simulink library "microCHP_modulating"  (R2018b)
settings: Solver=ode45  StartTime=0.0  StopTime=10.0  RelTol=1e-3  EnableMultiTasking=on
undefined symbols (not defined in the file): path_carnot
libraries: carnot x10
settings Model: Creator=lena.frank  LastModifiedBy=P41573
settings DataIOCC: LimitDataPoints=on  SaveFormat=Array  SignalLoggingSaveFormat=ModelDataLogs
settings OptimizationCC: ExpressionDepthLimit=2147483647  LifeSpan=inf
settings DebuggingCC: UnderspecifiedInitializationDetection=Classic  MergeDetectMultiDrivingBlocksExec=none  SolverPrmCheckMsg=warning  FcnCallInpInsideContextMsg=warning  StateNameClashWarn=warning  SFUnexpectedBacktrackingDiag=warning  SFNoUnconditionalDefaultTransitionDiag=warning  SFExecutionAtInitializationDiag=none
settings HardwareCC: ProdBitPerPointer=32  ProdBitPerSizeT=32  ProdBitPerPtrDiffT=32  ProdLargestAtomicFloat=None  ProdIntDivRoundTo=Undefined  ProdEndianess=Unspecified  ProdWordSize=32  ProdHWDeviceType=32-bit Generic
settings ModelReferenceCC: PropagateSignalLabelsOutOfModel=off
settings SFSimCC: SimUseLocalCustomCode=off
settings RTWCC: RTWUseLocalCustomCode=off
settings CodeAppCC: StateflowObjectComments=on
settings GRTTargetCC: TargetLangStandard=C89/C90 (ANSI)  GeneratePreprocessorConditionals=Disable all  CombineOutputUpdateFcns=off  GRTInterface=on
settings ConfigComp: CovMetricSettings=dw  CovHtmlReporting=on  CovSaveCumulativeToWorkspaceVar=on  CovSaveSingleToWorkspaceVar=on  CovExternalEMLEnable=off

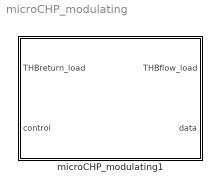
== system microCHP_modulating ==
  microCHP_modulating1 : Subsystem  mask(CHP){P_th_max=12500, P_th_min=3500, P_th_start=8000, f_P_el=0.37, T_flow_setpoint=80, T_flow_max=88, t_start=180, t_readjustment=450}
      mask prompts: P_th_max "maximum heating power [W]"; P_th_min "minimum heating power [W]"; P_th_start "initial heating power at start-up phase [W]"; f_P_el "electrical power fraction (referring to heating power) [0..1]"; T_flow_setpoint "flow setpoint temperature [°C]"; T_flow_max "maximum flow temperature [°C]"; t_start "duration of start-up phase [s]"; t_readjustment "duration of readjustment intervall [s]"
      mask help:
      | engine speed = f(T_return_load, T_flow_setpoint, T_flow, T_return)
      | T_return_load: a storage temperature or the return flow temperature.
      | Adjustable start-up phase: initial heating power
      | Ramp-up phase: maximum heating power up to 60°C
      | Control phase: heating power is readjusted after an inputed readjustment intervall.
      |
      | Return temperature raising facility.
      mask Help: eval('filetest (''manual.htm#electric_heating'')')
      mask Display: plot(0,0,100,100,[50,50,60,40,50],[55,40,70,60,90],[59,50],[48,40])

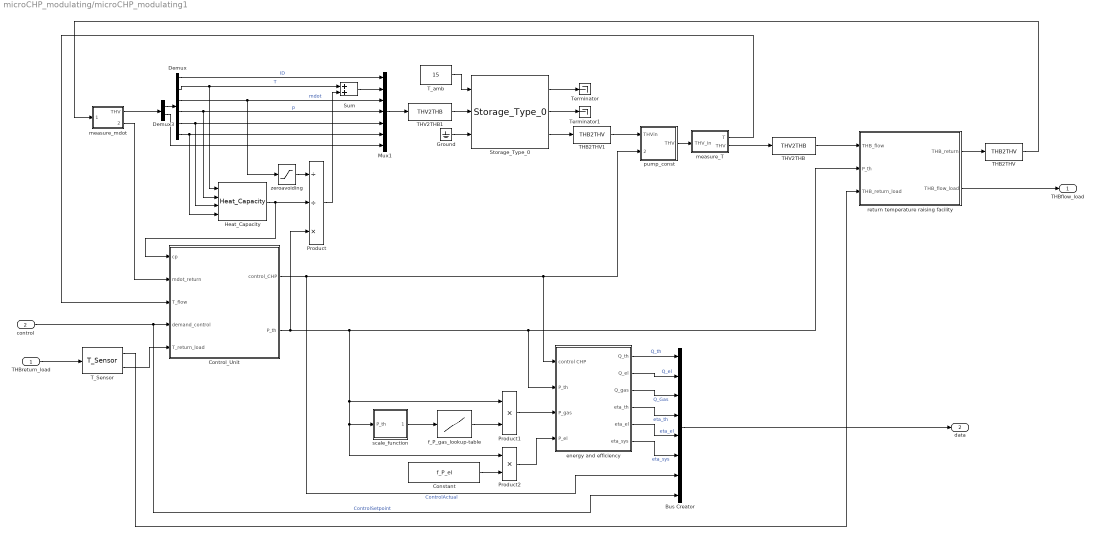
== system microCHP_modulating/microCHP_modulating1 ==
  THBreturn_load : Inport
  control : Inport  Port=2
  Bus Creator : BusCreator  Inputs=8
  Constant : Constant  Value=f_P_el
  Control_Unit : Subsystem
  Demux : Demux  Outputs=[1 1 1 1 1 1]
  Demux3 : Demux  Outputs=[6 14]
  Ground : Ground
  Heat_Capacity : carnot/Basic/Material_Properties/Heat_Capacity  VariantControl=CarlibClassic  INPUTARGUMENTS=state variables (classic)  DEBUGLEVEL=DEBUGLEVEL  MAXTOTALWARNINGS=inf  MAXCONSECUTIVEWARNINGS=inf  WRITETOFILE=0  FILENAME='errors.txt'
      settings: SourceProductName=Carnot
  Mux1 : Mux  Inputs=[1 1 1 1 1 1 14]
  Product : Product  Inputs=//*  SaturateOnIntegerOverflow=on  RndMeth=Zero  InputSameDT=on  OutDataTypeStr=Inherit: Same as first input
  Product1 : Product  Inputs=**  SaturateOnIntegerOverflow=on  RndMeth=Zero  InputSameDT=on  OutDataTypeStr=Inherit: Same as first input
  Product2 : Product  Inputs=**  SaturateOnIntegerOverflow=on  RndMeth=Zero  InputSameDT=on  OutDataTypeStr=Inherit: Same as first input
  Storage_Type_0 : carnot/Storage/Thermal/Storage_Type_0  t0=25  hgt=0.95493  stgtype=0  mpts=[1 2 3 4 5]  tini=[25 25 25 25 25]  PathName=fullfile(path_carnot('libsl'),'Storage','Thermal','Storage_Type_0','parameter_set')  FileName='<user defined>'  userPath=off  userParam=on  uwall=1  ubot=1  utop=1  axcond=1  volume=0.03  dia=0.2  standing=standing cylinder  nodes=5  mpoints=5  Tsensor=0.5  pipe1inlet=1  pipe1outlet=0  pipe1dia=0.03  heater1start=0.2  heater1end=0.25
      settings: SourceProductName=Carnot
  Sum : Sum  SaturateOnIntegerOverflow=on  InputSameDT=on  OutDataTypeStr=Inherit: Same as first input
  THB2THV : carnot/Toolbox/THB2THV
      settings: SourceProductName=Carnot
  THB2THV1 : carnot/Toolbox/THB2THV
      settings: SourceProductName=Carnot
  THV2THB : carnot/Toolbox/THV2THB
      settings: SourceProductName=Carnot
  THV2THB1 : carnot/Toolbox/THV2THB
      settings: SourceProductName=Carnot
  T_Sensor : carnot/Control/T_Sensor  tc=10  t0=20
      settings: SourceProductName=Carnot
  T_amb : Constant  Value=15
  Terminator : Terminator
  Terminator1 : Terminator
  energy and efficiency : Subsystem
  f_P_gas_lookup-table : Lookup_n-D  NumberOfTableDimensions=1  BreakpointsForDimension1=[1,2]  BreakpointsForDimension2=[44,80]  BreakpointsForDimension3=[1:2]  BreakpointsForDimension4=[1:2]  Table=[1.79 1.5]  InputSameDT=on
  measure_T : Subsystem  mask(temperature measurement sensor){tc=10, t0=25}
      mask prompts: tc "time constant of sensor [s]"; t0 "initial temperature [degree centigrade]"
      mask help: Measurement sensor for temperatures with first-oder hold. Temperature is in degree centigrade.
      mask init:
      | tc = 1/max(tc, 0.001);
      mask Help: eval('man (''measure_T'')')
      mask Display: plot(-18,0,30,20,[0 20],[0 0],[10 10 8 8 12 12 10],[0 8 8 17 17 8 8],[10 10 9 9 11 11 10 9],[15 10 10 9 9 10 9 10])
  measure_mdot : Subsystem  mask(massflow measurement sensor){}
      mask help: Measurement sensor for massflow in kg/s.
      mask Help: eval('man (''measure_mdot'')')
  pump_const : Subsystem  mask(constant pump){mdotmax=0.3, fluid_id=water, mix=0, dia=0.0157, power=100, p0=3e5}
      mask prompts: mdotmax "massflow rate [kg/s]"; fluid_id "fluid"; mix "percentage of fluid mix [0..1]"; dia "diameter at in- and outlet [m]"; power "electric power consumption [W]"; p0 "system pressure [Pa]"
      mask help: set constant massflow rate
      mask init:
      | mix = min(1, max(0, mix));
      | dia = max(0.001, dia);
      | p0 = max(p0, 1e5);
      mask Help: eval('man(''pump_const'')')
      mask TypeOptions fluid_id: water | air | cotton_oil | silicone_oil | water_glycol_mix
      mask Display: plot(0,0,100,100,[40,70,40,30,30,40,60,70,70,60,40],[70,50,30,40,60,70,70,60,40,30,30])
  return temperature raising facility : Subsystem  mask(return temperature raising facility){}
      mask help: A return setpoint temperature is calculated depending on heating power and flow setpoint temperature. The thermostatic mixer is located in the return flow of the CHP.
  scale_function : Subsystem
  zeroavoiding : Saturate  UpperLimit=inf  LowerLimit=1e-5
  THBflow_load : Outport
  data : Outport  Port=2
  wires:
  Storage_Type_0/1 -> Terminator/1
  T_amb/1 -> Storage_Type_0/1
  Storage_Type_0/3 -> THB2THV1/1
  THV2THB1/1 -> Storage_Type_0/2
  THV2THB/1 -> return temperature raising facility/1(THB_flow)
  THB2THV/1 -> measure_mdot/1(THV_in)
  control/1 -> Control_Unit/4(demand_control), Bus Creator/8  "ControlSetpoint"
  T_Sensor/1 -> return temperature raising facility/3(THB_return_load)
  return temperature raising facility/2(THB_flow_load) -> THBflow_load/1
  Bus Creator/1 -> data/1
  energy and efficiency/6(eta_sys) -> Bus Creator/6  "eta_sys"
  energy and efficiency/5(eta_el) -> Bus Creator/5  "eta_el"
  energy and efficiency/4(eta_th) -> Bus Creator/4  "eta_th"
  energy and efficiency/3(Q_gas) -> Bus Creator/3  "Q_Gas"
  energy and efficiency/2(Q_el) -> Bus Creator/2  "Q_el"
  energy and efficiency/1(Q_th) -> Bus Creator/1  "Q_th"
  Constant/1 -> Product2/2
  measure_mdot/1(THV) -> Demux3/1
  measure_T/2(THV) -> THV2THB/1
  return temperature raising facility/1(THB_return) -> THB2THV/1
  Product1/1 -> energy and efficiency/3(P_gas)
  f_P_gas_lookup-table/1 -> Product1/2
  Product2/1 -> energy and efficiency/4(P_el)
  scale_function/1(X_pth) -> f_P_gas_lookup-table/1
  Control_Unit/2(P_th) -> Product1/1, scale_function/1(P_th), Product2/1, energy and efficiency/2(P_th), return temperature raising facility/2(P_th), Product/3
  Control_Unit/1(control_CHP) -> energy and efficiency/1(control CHP), pump_const/2(control), Bus Creator/7  "ControlActual"
  pump_const/1(THV) -> measure_T/1(THV_in)
  THB2THV1/1 -> pump_const/1(THVin)
  zeroavoiding/1 -> Product/1
  measure_mdot/2(mdot) -> Control_Unit/2(mdot_return)
  measure_T/1(T) -> Control_Unit/3(T_flow)
  Heat_Capacity/1 -> Product/2, Control_Unit/1(cp)
  Demux/2 -> Sum/1, Heat_Capacity/1  "T"
  Product/1 -> Sum/2
  Mux1/1 -> THV2THB1/1
  Demux3/2 -> Mux1/7
  Demux3/1 -> Demux/1
  Sum/1 -> Mux1/2
  Demux/3 -> zeroavoiding/1, Mux1/3  "mdot"
  Demux/6 -> Heat_Capacity/4, Mux1/6
  Demux/5 -> Heat_Capacity/3, Mux1/5
  Demux/1 -> Mux1/1  "ID"
  Demux/4 -> Heat_Capacity/2, Mux1/4  "p"
  Storage_Type_0/2 -> Terminator1/1
  T_Sensor/2 -> Control_Unit/5(T_return_load)
  THBreturn_load/1 -> T_Sensor/1
  Ground/1 -> Storage_Type_0/3

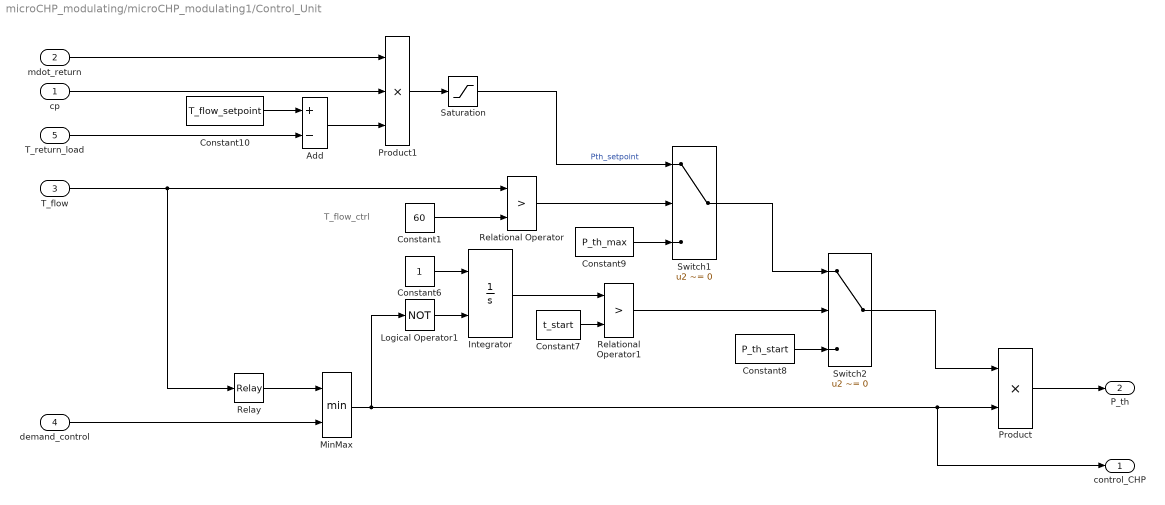
== system microCHP_modulating/microCHP_modulating1/Control_Unit ==
  note: T_flow_ctrl
  cp : Inport
  mdot_return : Inport  Port=2
  T_flow : Inport  Port=3
  demand_control : Inport  Port=4
  T_return_load : Inport  Port=5
  Add : Sum  Inputs=+-
  Constant1 : Constant  Value=60
  Constant10 : Constant  Value=T_flow_setpoint
  Constant6 : Constant
  Constant7 : Constant  Value=t_start
  Constant8 : Constant  Value=P_th_start
  Constant9 : Constant  Value=P_th_max
  Integrator : Integrator  ExternalReset=level
  Logical Operator1 : Logic  Operator=NOT  AllPortsSameDT=off  OutDataTypeStr=boolean
  MinMax : MinMax  Inputs=2
  Product : Product
  Product1 : Product  Inputs=3
  Relational Operator : RelationalOperator  Operator=>  OutDataTypeStr=boolean  RndMeth=Simplest
  Relational Operator1 : RelationalOperator  Operator=>  OutDataTypeStr=boolean  RndMeth=Simplest
  Relay : Relay  OnSwitchValue=T_flow_max  OffSwitchValue=T_flow_max-1  OnOutputValue=0  OffOutputValue=1
  Saturation : Saturate  UpperLimit=P_th_max  LowerLimit=P_th_min
  Switch1 : Switch  Criteria=u2 ~= 0
  Switch2 : Switch  Criteria=u2 ~= 0
  control_CHP : Outport
  P_th : Outport  Port=2
  wires:
  Switch2/1 -> Product/1
  Product1/1 -> Saturation/1
  Constant10/1 -> Add/1
  Switch1/1 -> Switch2/1
  Constant9/1 -> Switch1/3
  Constant8/1 -> Switch2/3
  Relational Operator1/1 -> Switch2/2
  Constant7/1 -> Relational Operator1/2
  Integrator/1 -> Relational Operator1/1
  Logical Operator1/1 -> Integrator/2
  Constant6/1 -> Integrator/1
  Saturation/1 -> Switch1/1  "Pth_setpoint"
  Relational Operator/1 -> Switch1/2
  Constant1/1 -> Relational Operator/2
  MinMax/1 -> Logical Operator1/1, Product/2, control_CHP/1
  Relay/1 -> MinMax/1
  Add/1 -> Product1/3
  T_flow/1 -> Relational Operator/1, Relay/1
  demand_control/1 -> MinMax/2
  mdot_return/1 -> Product1/1
  Product/1 -> P_th/1
  cp/1 -> Product1/2
  T_return_load/1 -> Add/2

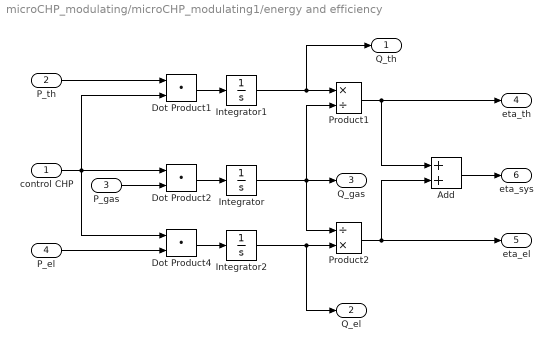
== system microCHP_modulating/microCHP_modulating1/energy and efficiency ==
  control CHP : Inport
  P_th : Inport  Port=2
  P_gas : Inport  Port=3
  P_el : Inport  Port=4
  Add : Sum
  Dot Product1 : DotProduct  InputSameDT=on  OutDataTypeStr=Inherit: Inherit via internal rule
  Dot Product2 : DotProduct  InputSameDT=on  OutDataTypeStr=Inherit: Inherit via internal rule
  Dot Product4 : DotProduct  InputSameDT=on  OutDataTypeStr=Inherit: Inherit via internal rule
  Integrator : Integrator
  Integrator1 : Integrator
  Integrator2 : Integrator
  Product1 : Product  Inputs=*/  SaturateOnIntegerOverflow=on  RndMeth=Zero  InputSameDT=on  OutDataTypeStr=Inherit: Same as first input
  Product2 : Product  Inputs=/*  SaturateOnIntegerOverflow=on  RndMeth=Zero  InputSameDT=on  OutDataTypeStr=Inherit: Same as first input
  Q_th : Outport
  Q_el : Outport  Port=2
  Q_gas : Outport  Port=3
  eta_th : Outport  Port=4
  eta_el : Outport  Port=5
  eta_sys : Outport  Port=6
  wires:
  Add/1 -> eta_sys/1
  Product1/1 -> eta_th/1, Add/1
  Integrator1/1 -> Q_th/1, Product1/1
  P_th/1 -> Dot Product1/1
  Dot Product1/1 -> Integrator1/1
  Integrator2/1 -> Q_el/1, Product2/2
  Integrator/1 -> Product1/2, Q_gas/1, Product2/1
  control CHP/1 -> Dot Product1/2, Dot Product4/1, Dot Product2/1
  Dot Product2/1 -> Integrator/1
  Dot Product4/1 -> Integrator2/1
  Product2/1 -> Add/2, eta_el/1
  P_el/1 -> Dot Product4/2
  P_gas/1 -> Dot Product2/2

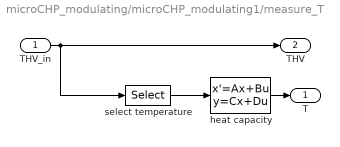
== system microCHP_modulating/microCHP_modulating1/measure_T ==
  THV_in : Inport
  heat capacity : StateSpace  A=-tc  B=tc  D=0  InitialCondition=t0
  select temperature : Selector  InputPortWidth=20  IndexOptions=Index vector (dialog)  Indices=[2]  OutputSizes=1
  T : Outport
  THV : Outport  Port=2
  wires:
  heat capacity/1 -> T/1
  select temperature/1 -> heat capacity/1
  THV_in/1 -> THV/1, select temperature/1

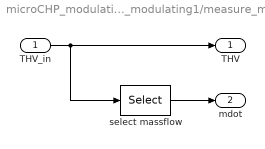
== system microCHP_modulating/microCHP_modulating1/measure_mdot ==
  THV_in : Inport
  select massflow : Selector  InputPortWidth=20  IndexOptions=Index vector (dialog)  Indices=[3]  OutputSizes=1
  THV : Outport
  mdot : Outport  Port=2
  wires:
  select massflow/1 -> mdot/1
  THV_in/1 -> THV/1, select massflow/1

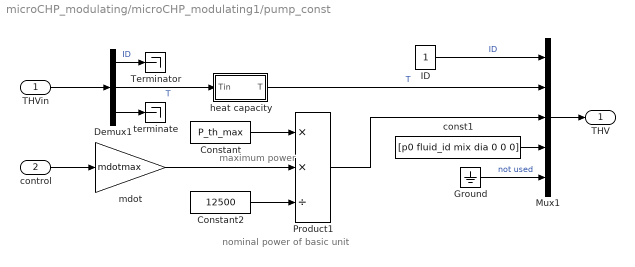
== system microCHP_modulating/microCHP_modulating1/pump_const ==
  note: nominal power of basic unit
  note: maximum power
  THVin : Inport
  control : Inport  Port=2
  Constant : Constant  Value=P_th_max
  Constant2 : Constant  Value=12500
  Demux1 : Demux  Outputs=[1 1 18]
  Ground : Ground
  ID : Constant
  Mux1 : Mux  Inputs=[1 1 1 7 10]
  Product1 : Product  Inputs=**/  SaturateOnIntegerOverflow=on  RndMeth=Zero  InputSameDT=on  OutDataTypeStr=Inherit: Same as first input
  Terminator : Terminator
  const1 : Constant  Value=[p0 fluid_id mix dia 0 0 0]
  heat capacity : Subsystem  mask{NTU=3.1}
      mask prompts: NTU "NTU (k*A/(m*cp))"
  mdot : Gain  Gain=mdotmax  SaturateOnIntegerOverflow=on  OutDataTypeStr=Inherit: Same as input  ParamDataTypeStr=Inherit: Same as input
  terminate : Terminator
  THV : Outport
  wires:
  control/1 -> mdot/1
  heat capacity/1(T) -> Mux1/2  "T"
  Product1/1 -> Mux1/3
  Constant2/1 -> Product1/3
  Constant/1 -> Product1/1
  mdot/1 -> Product1/2
  Demux1/2 -> heat capacity/1(Tin)  "T"
  Demux1/1 -> Terminator/1  "ID"
  const1/1 -> Mux1/4
  Mux1/1 -> THV/1
  ID/1 -> Mux1/1  "ID"
  THVin/1 -> Demux1/1
  Demux1/3 -> terminate/1
  Ground/1 -> Mux1/5  "not used"

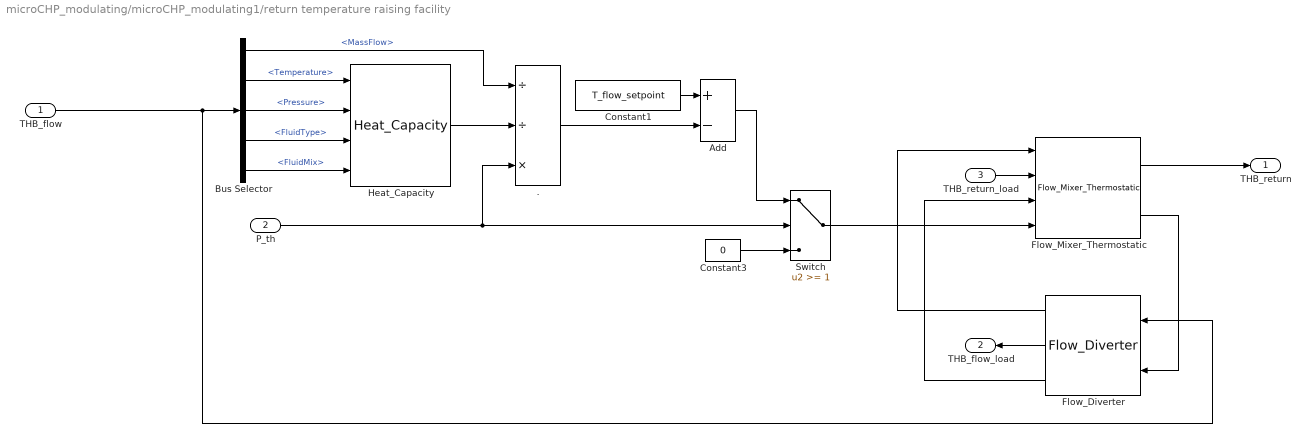
== system microCHP_modulating/microCHP_modulating1/return temperature raising facility ==
  THB_flow : Inport
  P_th : Inport  Port=2
  THB_return_load : Inport  Port=3
  . : Product  Inputs=//*  SaturateOnIntegerOverflow=on  RndMeth=Zero  InputSameDT=on  OutDataTypeStr=Inherit: Same as first input
  Add : Sum  Inputs=+-
  Bus Selector : BusSelector  OutputSignals=MassFlow,Temperature,Pressure,FluidType,FluidMix
  Constant1 : Constant  Value=T_flow_setpoint
  Constant3 : Constant  Value=0
  Flow_Diverter : carnot/Hydraulics/Flow_Diverter
      settings: SourceProductName=Carnot
  Flow_Mixer_Thermostatic : carnot/Hydraulics/Flow_Mixer_Thermostatic  t=1
      settings: SourceProductName=Carnot
  Heat_Capacity : carnot/Basic/Material_Properties/Heat_Capacity  VariantControl=CarlibClassic  INPUTARGUMENTS=state variables (classic)  DEBUGLEVEL=DEBUGLEVEL  MAXTOTALWARNINGS=inf  MAXCONSECUTIVEWARNINGS=inf  WRITETOFILE=0  FILENAME='errors.txt'
      settings: SourceProductName=Carnot
  Switch : Switch  Threshold=1  SaturateOnIntegerOverflow=on  InputSameDT=on
  THB_return : Outport
  THB_flow_load : Outport  Port=2
  wires:
  Flow_Diverter/3 -> Flow_Mixer_Thermostatic/3
  Flow_Diverter/1 -> Flow_Mixer_Thermostatic/1
  Flow_Mixer_Thermostatic/1 -> THB_return/1
  Flow_Mixer_Thermostatic/2 -> Flow_Diverter/2
  THB_flow/1 -> Bus Selector/1, Flow_Diverter/1
  Switch/1 -> Flow_Mixer_Thermostatic/4
  Constant3/1 -> Switch/3
  ./1 -> Add/2
  Add/1 -> Switch/1
  Constant1/1 -> Add/1
  THB_return_load/1 -> Flow_Mixer_Thermostatic/2
  Flow_Diverter/2 -> THB_flow_load/1
  Bus Selector/3 -> Heat_Capacity/2  "<Pressure>"
  Bus Selector/4 -> Heat_Capacity/3  "<FluidType>"
  Bus Selector/5 -> Heat_Capacity/4  "<FluidMix>"
  Bus Selector/1 -> ./1  "<MassFlow>"
  Bus Selector/2 -> Heat_Capacity/1  "<Temperature>"
  Heat_Capacity/1 -> ./2
  P_th/1 -> Switch/2, ./3

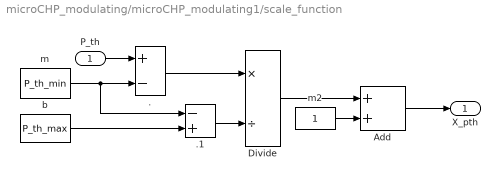
== system microCHP_modulating/microCHP_modulating1/scale_function ==
  P_th : Inport
  . : Sum  Inputs=+-
  .1 : Sum  Inputs=-+
  Add : Sum
  Divide : Product  Inputs=*/
  b : Constant  Value=P_th_max
  m : Constant  Value=P_th_min
  m2 : Constant
  X_pth : Outport
  wires:
  Add/1 -> X_pth/1
  Divide/1 -> Add/1
  P_th/1 -> ./1
  .1/1 -> Divide/2
  b/1 -> .1/2
  ./1 -> Divide/1
  m/1 -> .1/1, ./2
  m2/1 -> Add/2

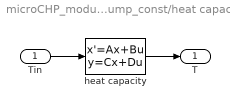
== system microCHP_modulating/microCHP_modulating1/pump_const/heat capacity ==
  Tin : Inport
  heat capacity : StateSpace  A=-NTU  B=NTU  D=0  InitialCondition=80
  T : Outport
  wires:
  Tin/1 -> heat capacity/1
  heat capacity/1 -> T/1
